simulink model "trajectory_planner"  (R2025a)
settings: configuration reference "MCConfiguration" (kept outside this file)
undefined symbols (not defined in the file): dspblkCoreblockFVToolHelper, gcbh
libraries: simulink x1
settings Model: DataDictionary=embeddedBoard_common.sldd  Creator=rpumpo  LastModifiedBy=rpumpo
settings ConfigSetRef: SourceName=MCConfiguration

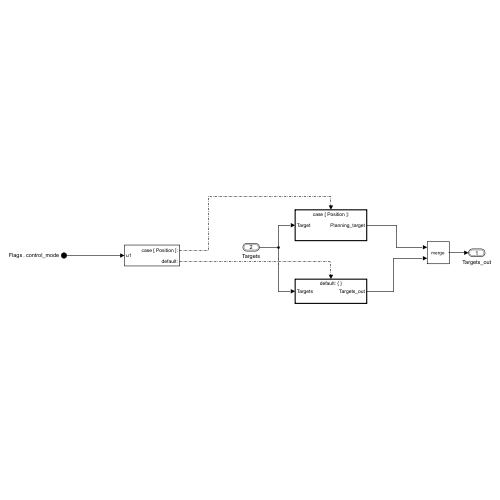
[thumbnail: Simulink's stored preview of the top-level diagram]
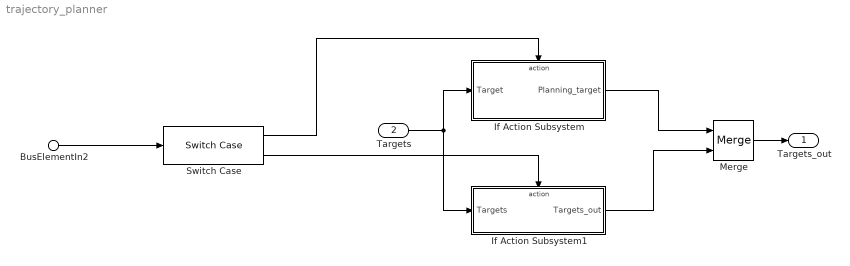
== system trajectory_planner ==
  BusElementIn2 : Inport  Description=control mode  PortName=Flags  Element=control_mode
  Targets : Inport  Port=2  OutDataTypeStr=Bus: Targets  BusOutputAsStruct=on
  If Action Subsystem : Subsystem  TreatAsAtomicUnit=on
  If Action Subsystem1 : Subsystem  TreatAsAtomicUnit=on
  Merge : Merge
  Switch Case : SwitchCase  CaseConditions={ControlModes.Position}
  Targets_out : Outport  OutDataTypeStr=Bus: Targets  BusOutputAsStruct=on
  wires:
  BusElementIn2/1 -> Switch Case/1
  Switch Case/1 -> If Action Subsystem/Action
  Switch Case/2 -> If Action Subsystem1/Action
  Targets/1 -> If Action Subsystem/1(Target), If Action Subsystem1/1(Targets)
  If Action Subsystem/1(Planning_target) -> Merge/1
  If Action Subsystem1/1(Targets_out) -> Merge/2
  Merge/1 -> Targets_out/1

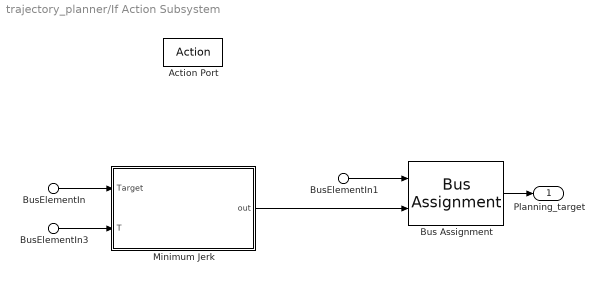
== system trajectory_planner/If Action Subsystem ==
  BusElementIn1 : Inport  PortName=Target
  BusElementIn3 : Inport  Description=Target time for position control  PortName=Target  Element=trajectory_time
  BusElementIn : Inport  PortName=Target  Element=position
  Action Port : ActionPort  ActionPortLabel=case [ Position ]:
  Bus Assignment : BusAssignment  AssignedSignals=position
  Minimum Jerk : Subsystem  mask{Ts=0.001}
      mask prompts: Ts "SampleTime"
  Planning_target : Outport  OutDataTypeStr=Bus: Targets  BusOutputAsStruct=on
  wires:
  Bus Assignment/1 -> Planning_target/1
  BusElementIn3/1 -> Minimum Jerk/2(T)
  BusElementIn1/1 -> Bus Assignment/1
  BusElementIn/1 -> Minimum Jerk/1(Target)
  Minimum Jerk/1(out) -> Bus Assignment/2

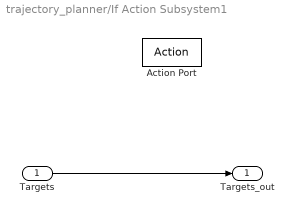
== system trajectory_planner/If Action Subsystem1 ==
  Targets : Inport  OutDataTypeStr=Bus: Targets
  Action Port : ActionPort  ActionPortLabel=default:
  Targets_out : Outport  OutDataTypeStr=Bus: Targets
  wires:
  Targets/1 -> Targets_out/1

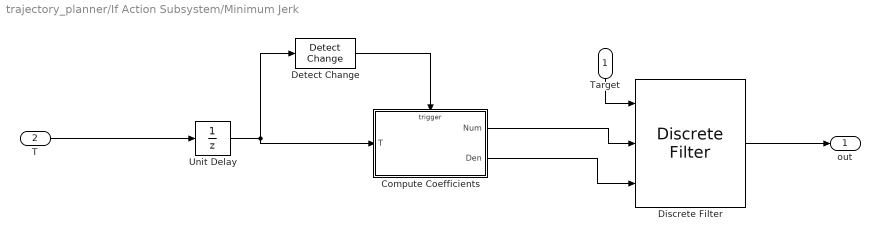
== system trajectory_planner/If Action Subsystem/Minimum Jerk ==
  Target : Inport  OutDataTypeStr=single  PortDimensions=1
  T : Inport  Port=2  OutDataTypeStr=single  PortDimensions=1
  Compute Coefficients : Subsystem  AncestorBlock=arsenal/Filters/Discrete Minimum Jerk/Compute Coefficients
  Detect Change : simulink/Logic and Bit Operations/Detect Change  vinit=0  OutDataTypeStr=uint8
  Discrete Filter : DiscreteFilter  LoadFcn=dspblkCoreblockFVToolHelper(gcbh,'load');  NumeratorSource=Input port  DenominatorSource=Input port  a0EqualsOne=on
      settings: CopyFcn=dspblkCoreblockFVToolHelper(gcbh,'copy');  DeleteFcn=dspblkCoreblockFVToolHelper(gcbh,'close');  ModelCloseFcn=dspblkCoreblockFVToolHelper(gcbh,'close');  PreSaveFcn=dspblkCoreblockFVToolHelper(gcbh,'presave');  PostSaveFcn=dspblkCoreblockFVToolHelper(gcbh,'postsave');  CloseFcn=dspblkCoreblockFVToolHelper(gcbh,'close');  InputPortMap=u0,p1,p3
  Unit Delay : UnitDelay  SampleTime=Ts  HasFrameUpgradeWarning=on
  out : Outport  OutDataTypeStr=single  PortDimensions=1
  wires:
  Discrete Filter/1 -> out/1
  Detect Change/1 -> Compute Coefficients/Trigger
  Target/1 -> Discrete Filter/1
  T/1 -> Unit Delay/1
  Unit Delay/1 -> Compute Coefficients/1(T), Detect Change/1
  Compute Coefficients/1(Num) -> Discrete Filter/2
  Compute Coefficients/2(Den) -> Discrete Filter/3

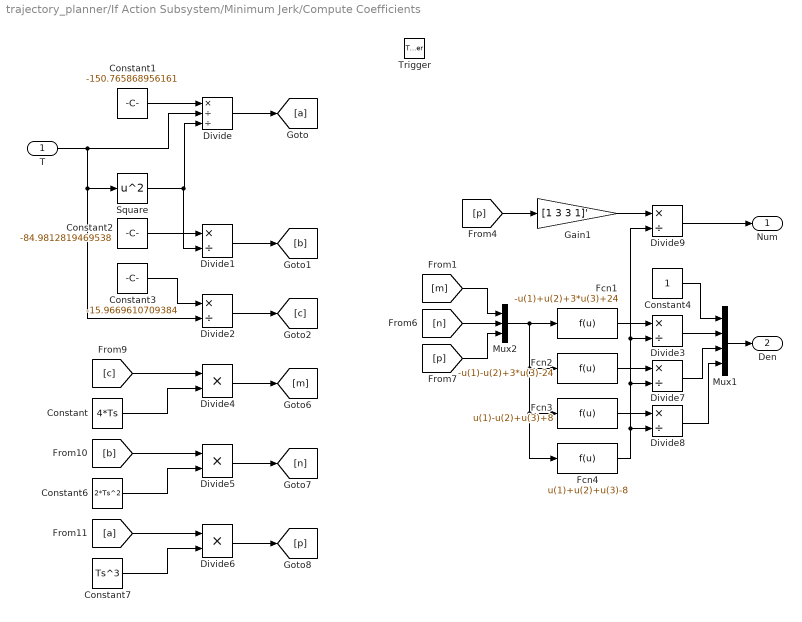
== system trajectory_planner/If Action Subsystem/Minimum Jerk/Compute Coefficients ==
  T : Inport
  Trigger : TriggerPort  VariantControl=(inherit)  PortDimensions=1
  Constant : Constant  Value=4*Ts  OutDataTypeStr=single
  Constant1 : Constant  Value=-150.765868956161  OutDataTypeStr=single
  Constant2 : Constant  Value=-84.9812819469538  OutDataTypeStr=single
  Constant3 : Constant  Value=-15.9669610709384  OutDataTypeStr=single
  Constant4 : Constant  OutDataTypeStr=single
  Constant6 : Constant  Value=2*Ts^2  OutDataTypeStr=single
  Constant7 : Constant  Value=Ts^3  OutDataTypeStr=single
  Divide : Product  Inputs=*//
  Divide1 : Product  Inputs=*/
  Divide2 : Product  Inputs=*/
  Divide3 : Product  Inputs=*/  OutDataTypeStr=single
  Divide4 : Product  Inputs=**
  Divide5 : Product  Inputs=**
  Divide6 : Product  Inputs=**
  Divide7 : Product  Inputs=*/  OutDataTypeStr=single
  Divide8 : Product  Inputs=*/  OutDataTypeStr=single
  Divide9 : Product  Inputs=*/
  Fcn1 : Fcn  Expr=-u(1)+u(2)+3*u(3)+24
  Fcn2 : Fcn  Expr=-u(1)-u(2)+3*u(3)-24
  Fcn3 : Fcn  Expr=u(1)-u(2)+u(3)+8
  Fcn4 : Fcn  Expr=u(1)+u(2)+u(3)-8
  Gain1 : Gain  Gain=[1 3 3 1]'
  Mux1 : Mux
  Mux2 : Mux  Inputs=3
  Square : Math  Operator=square
  Num : Outport  InitialOutput=[0 0 0 0]
  Den : Outport  Port=2  InitialOutput=[1 0 0 0]'
  wires:
  Constant1/1 -> Divide/1
  Divide1/1 -> [b]
  T/1 -> Divide2/2, Square/1, Divide/2
  Divide2/1 -> [c]
  [p] -> Gain1/1
  Constant2/1 -> Divide1/1
  Constant3/1 -> Divide2/1
  Square/1 -> Divide1/2, Divide/3
  Divide/1 -> [a]
  Constant4/1 -> Mux1/1
  Mux1/1 -> Den/1
  Divide4/1 -> [m]
  [c] -> Divide4/1
  Constant/1 -> Divide4/2
  Constant6/1 -> Divide5/2
  [b] -> Divide5/1
  Divide5/1 -> [n]
  Divide6/1 -> [p]
  [a] -> Divide6/1
  Constant7/1 -> Divide6/2
  [m] -> Mux2/1
  [n] -> Mux2/2
  [p] -> Mux2/3
  Mux2/1 -> Fcn4/1, Fcn3/1, Fcn2/1, Fcn1/1
  Fcn1/1 -> Divide3/1
  Divide3/1 -> Mux1/2
  Divide7/1 -> Mux1/3
  Divide8/1 -> Mux1/4
  Fcn2/1 -> Divide7/1
  Fcn3/1 -> Divide8/1
  Fcn4/1 -> Divide8/2, Divide7/2, Divide9/2, Divide3/2
  Gain1/1 -> Divide9/1
  Divide9/1 -> Num/1
